simulink model "deedemo4"  (Simulink 3.00)
settings: Solver=ode45  SolverMode=SingleTasking  StartTime=0.0  StopTime=159.9  RelTol=1e-3  AbsTol=1e-6
PreLoadFcn:
  | deedemi4
values from neighbouring files (symbols this model uses):
  c1 = .3    (= 0.3)    [deedemi4.m]
  k1 = 5    [deedemi4.m]
  k2 = 5    [deedemi4.m]
  m1 = 10    [deedemi4.m]
  m2 = 5    [deedemi4.m]
settings Model: SaveTime=off  SaveOutput=off  Creator=sanjai  LastModifiedBy=sanjai

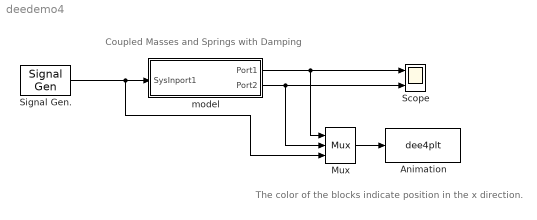
== system deedemo4 ==
  note: The color of the blocks indicate
      | position in the x direction.
  note: Coupled Masses and Springs with Damping
  Animation : S-Function  FunctionName=dee4plt  Parameters=1  PortCounts=[]  SFunctionModules=''
      settings: OpenFcn=global Handles; Handles = dee4plti;
      mask Display: disp('Animation')
  Mux : Mux  Inputs=3
      settings: DisplayOption=none
  Scope : Scope  NumInputPorts=2
      settings: TickLabels=on  TimeRange=60  YMin=-5~-5  YMax=5~5  SaveToWorkspace=off  SaveName=ScopeData  DataFormat=Matrix
  Signal Gen. : SignalGenerator  WaveForm=sine  Amplitude=2.000000  Frequency=4.860000  Units=rad/sec
  model : Subsystem
      settings: OpenFcn=diffeqed
      mask Type: Differential Equation Editor (DEE)
      mask Display: disp('damped \nmass/spring\n  system')
  wires:
  Signal Gen./1 -> Mux/3, model/1(SysInport1)
  model/2(Port2) -> Mux/2, Scope/2
  model/1(Port1) -> Mux/1, Scope/1
  Mux/1 -> Animation/1

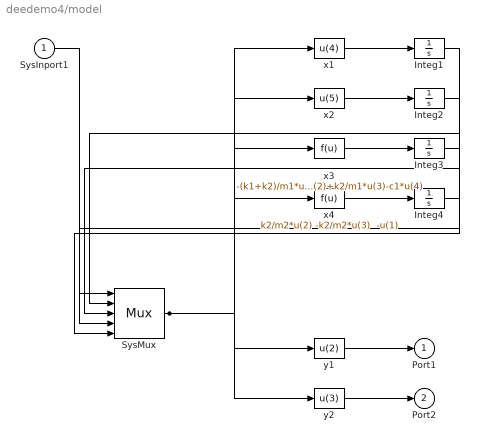
== system deedemo4/model ==
  SysInport1 : Inport  Port=1  PortWidth=-1  SampleTime=-1  DataType=auto
      settings: SignalType=auto
  Integ1 : Integrator  ExternalReset=none  InitialConditionSource=internal  InitialCondition=0  LimitOutput=off  UpperSaturationLimit=inf  LowerSaturationLimit=-inf  ShowSaturationPort=off  ShowStatePort=off  AbsoluteTolerance=auto
  Integ2 : Integrator  ExternalReset=none  InitialConditionSource=internal  InitialCondition=1.5  LimitOutput=off  UpperSaturationLimit=inf  LowerSaturationLimit=-inf  ShowSaturationPort=off  ShowStatePort=off  AbsoluteTolerance=auto
  Integ3 : Integrator  ExternalReset=none  InitialConditionSource=internal  InitialCondition=1.5  LimitOutput=off  UpperSaturationLimit=inf  LowerSaturationLimit=-inf  ShowSaturationPort=off  ShowStatePort=off  AbsoluteTolerance=auto
  Integ4 : Integrator  ExternalReset=none  InitialConditionSource=internal  InitialCondition=0  LimitOutput=off  UpperSaturationLimit=inf  LowerSaturationLimit=-inf  ShowSaturationPort=off  ShowStatePort=off  AbsoluteTolerance=auto
  SysMux : Mux  Inputs=5
      settings: DisplayOption=none
  x1 : Fcn  Expr=u(4)
  x2 : Fcn  Expr=u(5)
  x3 : Fcn  Expr=-(k1+k2)/m1*u(2)+k2/m1*u(3)-c1*u(4)
  x4 : Fcn  Expr="k2/m2*u(2) -k2/m2*u(3)  -u(1)"
  y1 : Fcn  Expr=u(2)
  y2 : Fcn  Expr=u(3)
  Port1 : Outport  Port=1  InitialOutput=0
  Port2 : Outport  Port=2  InitialOutput=0
  wires:
  y2/1 -> Port2/1
  SysMux/1 -> y2/1, y1/1, x4/1, x3/1, x2/1, x1/1
  y1/1 -> Port1/1
  Integ4/1 -> SysMux/5
  x4/1 -> Integ4/1
  Integ3/1 -> SysMux/4
  x3/1 -> Integ3/1
  Integ2/1 -> SysMux/3
  x2/1 -> Integ2/1
  Integ1/1 -> SysMux/2
  x1/1 -> Integ1/1
  SysInport1/1 -> SysMux/1
